simulink model "CTRL_LO_ST1_YAWTRQLATDIST_test"  (R2023b)
settings: Solver=VariableStepAuto  StartTime=0.0  StopTime=10.0  RelTol=1e-3
libraries: CTRL_LO_ST1_YAWTRQLATDIST x1
settings Model: Creator=blatak  LastModifiedBy=blatak

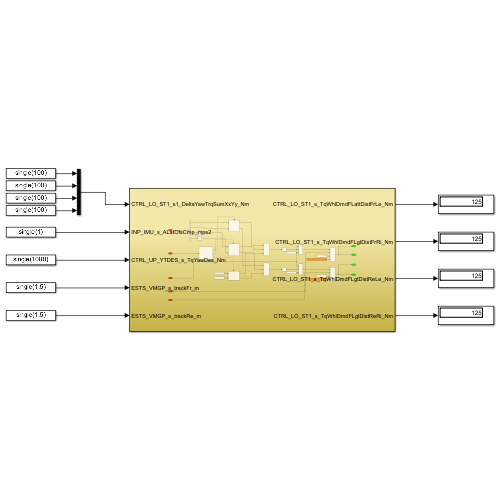
[thumbnail: Simulink's stored preview of the top-level diagram]
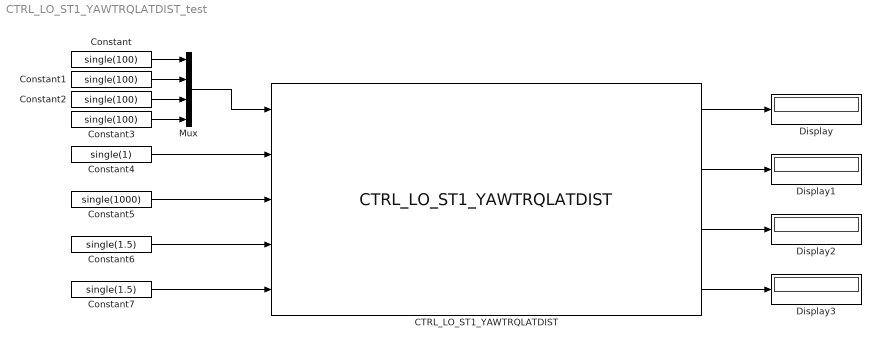
== system CTRL_LO_ST1_YAWTRQLATDIST_test ==
  CTRL_LO_ST1_YAWTRQLATDIST : CTRL_LO_ST1_YAWTRQLATDIST/CTRL_LO_ST1_YAWTRQLATDIST  SystemSampleTime=-1  VariantActivationTime=update diagram  AllowFlexibleInterface=on  Latency=0  AutoFrameSizeCalculation=off
  Constant{,1..3} (4 alike) : Constant  Value=single(100)
  Constant4 : Constant  Value=single(1)
  Constant5 : Constant  Value=single(1000)
  Constant6 : Constant  Value=single(1.5)
  Constant7 : Constant  Value=single(1.5)
  Display{,1..3} (4 alike) : Display
  Mux : Mux
  wires:
  Constant7/1 -> CTRL_LO_ST1_YAWTRQLATDIST/5
  Constant4/1 -> CTRL_LO_ST1_YAWTRQLATDIST/2
  Constant5/1 -> CTRL_LO_ST1_YAWTRQLATDIST/3
  Constant6/1 -> CTRL_LO_ST1_YAWTRQLATDIST/4
  Constant/1 -> Mux/1
  Constant1/1 -> Mux/2
  Constant2/1 -> Mux/3
  Constant3/1 -> Mux/4
  Mux/1 -> CTRL_LO_ST1_YAWTRQLATDIST/1
  CTRL_LO_ST1_YAWTRQLATDIST/1 -> Display/1
  CTRL_LO_ST1_YAWTRQLATDIST/2 -> Display1/1
  CTRL_LO_ST1_YAWTRQLATDIST/3 -> Display2/1
  CTRL_LO_ST1_YAWTRQLATDIST/4 -> Display3/1
